simulink model "SB8_discrete_done"  (R2024b)
settings: Solver=FixedStepDiscrete  StartTime=0.0  StopTime=10  FixedStep=0.05  RelTol=1e-3
undefined symbols (not defined in the file or in its folder): DiscIntNeverNeededParam
settings Model: Creator=admin  LastModifiedBy=admin

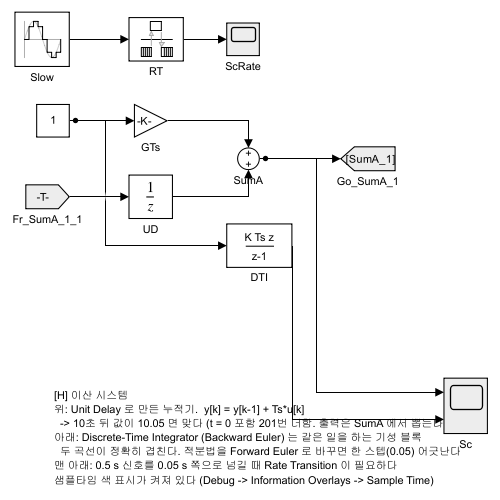
[thumbnail: Simulink's stored preview of the top-level diagram]
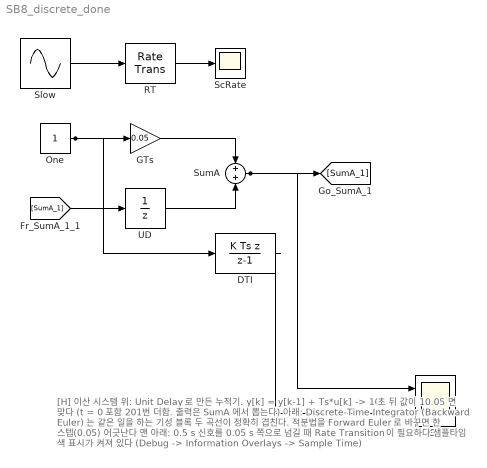
== system SB8_discrete_done ==
  note: [H] 이산 시스템
      | 위: Unit Delay 로 만든 누적기.  y[k] = y[k-1] + Ts*u[k]
      |   -> 10초 뒤 값이 10.05 면 맞다 (t = 0 포함 201번 더함. 출력은 SumA 에서 뽑는다)
      | 아래: Discrete-Time Integrator (Backward Euler) 는 같은 일을 하는 기성 블록
      |   두 곡선이 정확히 겹친다. 적분법을 Forward Euler 로 바꾸면 한 스텝(0.05) 어긋난다
      | 맨 아래: 0.5 s 신호를 0.05 s 쪽으로 넘길 때 Rate Transition 이 필요하다
      | 샘플타임 색 표시가 켜져 있다 (Debug -> Information Overlays -> Sample Time)
  DTI : DiscreteIntegrator  IntegratorMethod=Integration: Backward Euler  SampleTime=0.05  ICPrevOutput=DiscIntNeverNeededParam  ICPrevScaledInput=DiscIntNeverNeededParam
  GTs : Gain  Gain=0.05
  One : Constant
  RT : RateTransition  OutPortSampleTime=0.05
  Sc : Scope  NumInputPorts=2
  ScRate : Scope
  Slow : Sin  SampleTime=0.5
  SumA : Sum
  UD : UnitDelay  SampleTime=0.05  HasFrameUpgradeWarning=on
  wires:
  [SumA_1] -> UD/1
  Slow/1 -> RT/1
  One/1 -> DTI/1, GTs/1
  RT/1 -> ScRate/1
  GTs/1 -> SumA/1
  UD/1 -> SumA/2
  SumA/1 -> [SumA_1], Sc/1
  DTI/1 -> Sc/2
